simulink model "adc_to_10gbe"  (Simulink 7.4)
settings: Solver=ode45  StartTime=0.0  StopTime=200000  RelTol=1e-3
undefined symbols (not defined in the file): ROACH
libraries: xbsIndex_r4 x112, xps_library x77, casper_library_misc x6, xbsReplacements_r4 x3
(part 1 of 2)
settings Model: Creator=jkocz  LastModifiedBy=danny
settings OptimizationCC: InitFltsAndDblsToZero=on
settings DebuggingCC: SaveWithParameterizedLinksMsg=none  SignalResolutionControl=TryResolveAllWithWarning  MultiTaskDSMMsg=warning  MultiTaskCondExecSysMsg=none  StrictBusMsg=None
settings RTWCC: IncludeERTFirstTime=on
settings GRTTargetCC: TargetFcnLib=ansi_tfl_tmw.mat

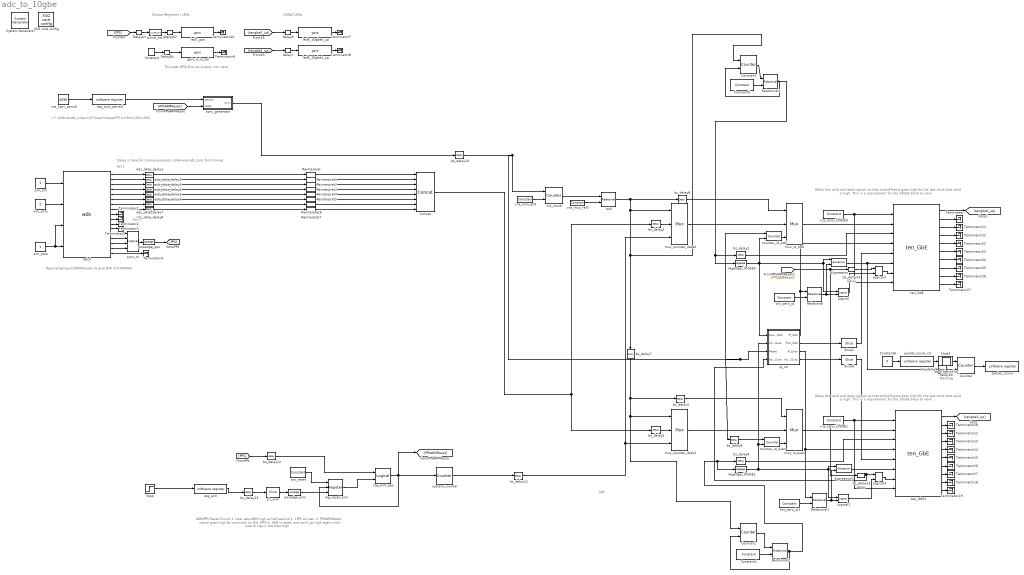
== system adc_to_10gbe ==
  note: left
  note: n * LCM(reoder_order=2)*(taps*clksperFFT=2*64=128)=256
  note: Pol 1
  note: Pol 2
  note: Real sampling at 800MSa/sec
      | to give B/W of 0-400MHz
  note: ARM/PPS Reset Circuit
      | 1. User sets ARM high at half-second
      | 2. 1PPS arrives.
      | 3. PPSARMReset signal goes high for one clock on the 1PPS
      | 4. ARM is reset, and won't go high again until user brings it low then high
  note: Delay is here for timing purposes:
      | otherwise adc_sync fails timing.
  note: Delay the valid and data signals so that
      | end-of-frame goes high for the last clock
      | that valid is high. This is a requirement for
      | the 10GbE block to work.
  note: Delay the valid and data signals so that
      | end-of-frame goes high for the last clock
      | that valid is high. This is a requirement for
      | the 10GbE block to work.
  note: This sets GPIO B as an output, not input
  note: Output Registers / LEDs
  note: 10GbE LEDa
  " System Generator" : xbsIndex_r4/ System Generator  Tag=genX  SystemSampleTime=-1  xilinxfamily=virtex2p  part=xc2vp50  speed=-7  package=ff1152  synthesis_tool=XST  clock_wrapper=Clock Enables  directory=./adc_to_10gbe_mod/sysgen  testbench=off  simulink_period=1  sysclk_period=5  dcm_input_clock_period=100  incr_netlist=off  trim_vbits=Everywhere in SubSystem  dbl_ovrd=According to Block Masks  core_generation=According to Block Masks  run_coregen=off  deprecated_control=off  eval_field=0  block_type=sysgen
      settings: block_version=10.1
  Concat : xbsIndex_r4/Concat  num_inputs=8  dbl_ovrd=off  block_type=concat
  Constant : xbsIndex_r4/Constant  arith_type=Boolean  const=0  n_bits=16  bin_pt=14  explicit_period=on  period=1  equ=P=C  opselect=C  inp2=PCIN>>17  opr=+  inp1=P  carry=CIN  dbl_ovrd=off  block_type=constant
      settings: block_version=11.4
  Constant1 : xbsIndex_r4/Constant  arith_type=Unsigned  const=1026  n_bits=11  bin_pt=0  explicit_period=off  period=1  equ=P=C  opselect=C  inp2=PCIN>>17  opr=+  inp1=P  carry=CIN  dbl_ovrd=off  block_type=constant
      settings: block_version=9.1.01
  Constant5 : xbsIndex_r4/Constant  arith_type=Unsigned  const=1026  n_bits=11  bin_pt=0  explicit_period=off  period=1  equ=P=C  opselect=C  inp2=PCIN>>17  opr=+  inp1=P  carry=CIN  dbl_ovrd=off  block_type=constant
      settings: block_version=9.1.01
  Constant6 : Constant  Value=0  OutDataType=sfix(16)  OutScaling=2^0
  Counter : xbsIndex_r4/Counter  cnt_type=Free Running  cnt_to=Inf  operation=Up  start_count=0  cnt_by_val=1  arith_type=Unsigned  n_bits=32  bin_pt=0  load_pin=off  rst=on  en=on  explicit_period=off  period=1  dbl_ovrd=off  use_behavioral_HDL=off  implementation=Fabric  use_rpm=on  block_type=counter
      settings: xl_area=[0, 0, 0, 0, 0, 0, 0]  block_version=10.1
  Counter1 : xbsIndex_r4/Counter  cnt_type=Free Running  cnt_to=1023  operation=Up  start_count=0  cnt_by_val=1  arith_type=Unsigned  n_bits=12  bin_pt=0  load_pin=off  rst=on  en=on  explicit_period=on  period=1  dbl_ovrd=off  use_behavioral_HDL=off  implementation=Fabric  use_rpm=on  block_type=counter
      settings: xl_area=[0, 0, 0, 0, 0, 0, 0]  block_version=9.1.01
  Counter3 : xbsIndex_r4/Counter  cnt_type=Free Running  cnt_to=1023  operation=Up  start_count=0  cnt_by_val=1  arith_type=Unsigned  n_bits=12  bin_pt=0  load_pin=off  rst=on  en=on  explicit_period=on  period=1  dbl_ovrd=off  use_behavioral_HDL=off  implementation=Fabric  use_rpm=on  block_type=counter
      settings: xl_area=[0, 0, 0, 0, 0, 0, 0]  block_version=9.1.01
  Delay{6..7,62..64} (5 alike) : xbsIndex_r4/Delay  en=off  latency=2  dbl_ovrd=off  reg_retiming=on  block_type=delay
  Expression : xbsIndex_r4/Expression  expression=a & ~b  align_bp=on  en=off  latency=0  precision=Full  arith_type=Unsigned  n_bits=8  bin_pt=2  dbl_ovrd=off  block_type=expr
      settings: xl_area=[0, 0, 0, 0, 0, 0, 0]  block_version=10.1
  Expression1 : xbsIndex_r4/Expression  expression=a & ~b  align_bp=on  en=off  latency=0  precision=Full  arith_type=Unsigned  n_bits=8  bin_pt=2  dbl_ovrd=off  block_type=expr
      settings: xl_area=[0, 0, 0, 0, 0, 0, 0]  block_version=10.1
  Logical : xbsIndex_r4/Logical  logical_function=AND  inputs=2  en=off  latency=0  precision=Full  arith_type=Unsigned  n_bits=8  bin_pt=2  align_bp=on  dbl_ovrd=off  block_type=logical
      settings: xl_area=[0, 0, 0, 0, 0, 0, 0]  block_version=10.1
  Logical1 : xbsIndex_r4/Logical  logical_function=AND  inputs=2  en=off  latency=0  precision=Full  arith_type=Unsigned  n_bits=8  bin_pt=2  align_bp=on  dbl_ovrd=off  block_type=logical
      settings: xl_area=[0, 0, 0, 0, 0, 0, 0]  block_version=10.1
  Logical3 : xbsIndex_r4/Logical  logical_function=OR  inputs=2  en=off  latency=0  precision=Full  arith_type=Unsigned  n_bits=8  bin_pt=2  align_bp=on  dbl_ovrd=off  block_type=logical
      settings: xl_area=[0, 0, 0, 0, 0, 0, 0]  block_version=10.1
  Logical4 : xbsIndex_r4/Logical  logical_function=OR  inputs=2  en=off  latency=0  precision=Full  arith_type=Unsigned  n_bits=8  bin_pt=2  align_bp=on  dbl_ovrd=off  block_type=logical
      settings: xl_area=[0, 0, 0, 0, 0, 0, 0]  block_version=10.1
  Reinterpret{,1..7} (8 alike) : xbsIndex_r4/Reinterpret  force_arith_type=on  arith_type=Unsigned  force_bin_pt=on  bin_pt=0  block_type=reinterpret
      Reinterpret settings: infoedit="Changes signal type without altering the binary representation.   You can changed the signal between signed and unsigned, and relocate the binary point.<br><br>Hardware notes: In hardware this block costs nothing.<br><br>Example:  Suppose the input is 6 bits wide, signed, with 2 fractional bits, and the output is forced to unsigned with 0 fractional bits.  Then an input of -2.0 (1110.00 in binary 2's complement) becomes an output of 56 (111000 in binary)."  block_version=10.1
      Reinterpret1 settings: infoedit="Changes signal type without altering the binary representation.   You can changed the signal between signed and unsigned, and relocate the binary point.<P><P>Hardware notes: In hardware this block costs nothing.<P><P>Example:  Suppose the input is 6 bits wide, signed, with 2 fractional bits, and the output is forced to unsigned with 0 fractional bits.  Then an input of -2.0 (1110.00 in binary 2's complement) becomes an output of 56 (111000 in binary)."  block_version=10.1
      Reinterpret2 settings: infoedit="Changes signal type without altering the binary representation.   You can changed the signal between signed and unsigned, and relocate the binary point.<P><P>Hardware notes: In hardware this block costs nothing.<P><P>Example:  Suppose the input is 6 bits wide, signed, with 2 fractional bits, and the output is forced to unsigned with 0 fractional bits.  Then an input of -2.0 (1110.00 in binary 2's complement) becomes an output of 56 (111000 in binary)."  block_version=10.1
      Reinterpret3 settings: infoedit="Changes signal type without altering the binary representation.   You can changed the signal between signed and unsigned, and relocate the binary point.<P><P>Hardware notes: In hardware this block costs nothing.<P><P>Example:  Suppose the input is 6 bits wide, signed, with 2 fractional bits, and the output is forced to unsigned with 0 fractional bits.  Then an input of -2.0 (1110.00 in binary 2's complement) becomes an output of 56 (111000 in binary)."  block_version=10.1
      Reinterpret4 settings: infoedit="Changes signal type without altering the binary representation.   You can changed the signal between signed and unsigned, and relocate the binary point.<P><P>Hardware notes: In hardware this block costs nothing.<P><P>Example:  Suppose the input is 6 bits wide, signed, with 2 fractional bits, and the output is forced to unsigned with 0 fractional bits.  Then an input of -2.0 (1110.00 in binary 2's complement) becomes an output of 56 (111000 in binary)."  block_version=10.1
      Reinterpret5 settings: infoedit="Changes signal type without altering the binary representation.   You can changed the signal between signed and unsigned, and relocate the binary point.<P><P>Hardware notes: In hardware this block costs nothing.<P><P>Example:  Suppose the input is 6 bits wide, signed, with 2 fractional bits, and the output is forced to unsigned with 0 fractional bits.  Then an input of -2.0 (1110.00 in binary 2's complement) becomes an output of 56 (111000 in binary)."  block_version=10.1
      Reinterpret6 settings: infoedit="Changes signal type without altering the binary representation.   You can changed the signal between signed and unsigned, and relocate the binary point.<P><P>Hardware notes: In hardware this block costs nothing.<P><P>Example:  Suppose the input is 6 bits wide, signed, with 2 fractional bits, and the output is forced to unsigned with 0 fractional bits.  Then an input of -2.0 (1110.00 in binary 2's complement) becomes an output of 56 (111000 in binary)."  block_version=10.1
      Reinterpret7 settings: infoedit="Changes signal type without altering the binary representation.   You can changed the signal between signed and unsigned, and relocate the binary point.<P><P>Hardware notes: In hardware this block costs nothing.<P><P>Example:  Suppose the input is 6 bits wide, signed, with 2 fractional bits, and the output is forced to unsigned with 0 fractional bits.  Then an input of -2.0 (1110.00 in binary 2's complement) becomes an output of 56 (111000 in binary)."  block_version=10.1
  Relational : xbsIndex_r4/Relational  mode=a=b  en=off  latency=1  dbl_ovrd=off  block_type=relational
      settings: xl_area=[0, 0, 0, 0, 0, 0, 0]  block_version=10.1
  Relational1 : xbsIndex_r4/Relational  mode=a=b  en=off  latency=1  dbl_ovrd=off  block_type=relational
      settings: xl_area=[0, 0, 0, 0, 0, 0, 0]  block_version=10.1
  Relational2 : xbsIndex_r4/Relational  mode=a!=b  en=off  latency=0  dbl_ovrd=off  block_type=relational
      settings: xl_area=[0, 0, 0, 0, 0, 0, 0]  block_version=9.1.01
  Relational5 : xbsIndex_r4/Relational  mode=a!=b  en=off  latency=0  dbl_ovrd=off  block_type=relational
      settings: xl_area=[0, 0, 0, 0, 0, 0, 0]  block_version=9.1.01
  Slice1 : xbsIndex_r4/Slice  nbits=16  boolean_output=off  mode=Lower Bit Location + Width  bit1=0  base1=MSB of Input  bit0=0  base0=LSB of Input  dbl_ovrd=off  block_type=slice
      settings: infoedit="Extracts a given range of bits from each input sample and presents it at the output.  The output type is ordinarily unsigned with binary point at zero, but can be Boolean when the slice is one bit wide.<P><P>Hardware notes: In hardware this block costs nothing."  block_version=10.1
  Slice3 : xbsIndex_r4/Slice  nbits=1  boolean_output=on  mode=Lower Bit Location + Width  bit1=0  base1=MSB of Input  bit0=0  base0=LSB of Input  dbl_ovrd=off  block_type=slice
      settings: infoedit="Extracts a given range of bits from each input sample and presents it at the output.  The output type is ordinarily unsigned with binary point at zero, but can be Boolean when the slice is one bit wide.<P><P>Hardware notes: In hardware this block costs nothing."  block_version=10.1
  Slice6 : xbsIndex_r4/Slice  nbits=16  boolean_output=off  mode=Lower Bit Location + Width  bit1=0  base1=MSB of Input  bit0=0  base0=LSB of Input  dbl_ovrd=off  block_type=slice
      settings: infoedit="Extracts a given range of bits from each input sample and presents it at the output.  The output type is ordinarily unsigned with binary point at zero, but can be Boolean when the slice is one bit wide.<P><P>Hardware notes: In hardware this block costs nothing."  block_version=10.1
  Step : Step  SampleTime=0
  Terminator{,1..5,7..9,11..28} (27 alike) : Terminator
  XSG core config : xps_library/XSG core config  Tag=xps:xsg  SystemSampleTime=-1  hw_sys=ROACH:sx95t  ibob_linux=off  clk_src=adc0_clk  iBOB_clk_src=adc0_clk  BEE2_ctrl_clk_src=sys_clk  BEE2_usr_clk_src=sys_clk  ROACH_clk_src=adc0_clk  CORR_clk_src=sys_clk  gpio_clk_io_group=iBOB:sma  gpio_clk_bit_index=0  clk_rate=100  sample_period=1  synthesis_tool=XST  mpc_type=powerpc440_ext
  adc0 : xps_library/adc  Tag=xps:adc  SystemSampleTime=-1  adc_brd=adc0  adc_clk_rate=800  adc_interleave=off  sample_period=1
  adc_data_delay{1..8} (8 alike) : xbsIndex_r4/Delay  en=off  latency=1  dbl_ovrd=off  reg_retiming=on  block_type=delay
      settings: xl_area=[0, 0, 0, 0, 0, 0, 0]  block_version=10.1
  bs_delay{1..2,4..5} (4 alike) : xbsIndex_r4/Delay  en=off  latency=1  dbl_ovrd=off  reg_retiming=off  block_type=delay
      settings: xl_area=[0, 0, 0, 0, 0, 0, 0]  block_version=10.1
  bs_delay{10..13} (4 alike) : xbsIndex_r4/Delay  en=off  latency=0  dbl_ovrd=off  reg_retiming=off  block_type=delay
      settings: xl_area=[0, 0, 0, 0, 0, 0, 0]  block_version=10.1
  bs_delay14 : xbsIndex_r4/Delay  en=off  latency=3  dbl_ovrd=off  reg_retiming=off  block_type=delay
      settings: xl_area=[0, 0, 0, 0, 0, 0, 0]  block_version=10.1
  bs_delay15 : xbsIndex_r4/Delay  en=off  latency=1027  dbl_ovrd=off  reg_retiming=off  block_type=delay
      settings: xl_area=[0, 0, 0, 0, 0, 0, 0]  block_version=10.1
  bs_delay3 : xbsIndex_r4/Delay  en=off  latency=2  dbl_ovrd=off  reg_retiming=off  block_type=delay
      settings: xl_area=[0, 0, 0, 0, 0, 0, 0]  block_version=10.1
  bs_delay6 : xbsIndex_r4/Delay  en=off  latency=4  dbl_ovrd=off  reg_retiming=off  block_type=delay
      settings: xl_area=[0, 0, 0, 0, 0, 0, 0]  block_version=10.1
  bs_delay7 : xbsIndex_r4/Delay  en=off  latency=1024  dbl_ovrd=off  reg_retiming=off  block_type=delay
      settings: xl_area=[0, 0, 0, 0, 0, 0, 0]  block_version=10.1
  bs_delay8 : xbsIndex_r4/Delay  en=off  latency=2  dbl_ovrd=off  reg_retiming=off  block_type=delay
      settings: xl_area=[0, 0, 0, 0, 0, 0, 0]  block_version=10.1
  bs_delay9 : xbsIndex_r4/Delay  en=off  latency=5  dbl_ovrd=off  reg_retiming=on  block_type=delay
      settings: xl_area=[0, 0, 0, 0, 0, 0, 0]  block_version=10.1
  cns_mux_en0 : xbsIndex_r4/Constant  arith_type=Boolean  const=1  n_bits=1  bin_pt=0  explicit_period=on  period=1  equ=P=C  opselect=C  inp2=PCIN>>17  opr=+  inp1=P  carry=CIN  dbl_ovrd=off  block_type=constant
      settings: block_version=10.1
  cns_mux_rel0 : xbsIndex_r4/Constant  arith_type=Unsigned  const=0  n_bits=11  bin_pt=0  explicit_period=on  period=1  equ=P=C  opselect=C  inp2=PCIN>>17  opr=+  inp1=P  carry=CIN  dbl_ovrd=off  block_type=constant
      settings: block_version=10.1
  cns_reset : xbsIndex_r4/Constant  arith_type=Boolean  const=1  n_bits=1  bin_pt=0  explicit_period=on  period=1  equ=P=C  opselect=C  inp2=PCIN>>17  opr=+  inp1=P  carry=CIN  dbl_ovrd=off  block_type=constant
      settings: block_version=10.1
  cns_sync_period : Constant  Value=4096  OutDataType=sfix(16)  OutScaling=2^0
  cns_zero_10GbE0 : xbsIndex_r4/Constant  arith_type=Boolean  const=0  n_bits=32  bin_pt=0  explicit_period=on  period=1  equ=P=C  opselect=C  inp2=PCIN>>17  opr=+  inp1=P  carry=CIN  dbl_ovrd=off  block_type=constant
      settings: block_version=10.1
  cns_zero_10GbE1 : xbsIndex_r4/Constant  arith_type=Boolean  const=0  n_bits=32  bin_pt=0  explicit_period=on  period=1  equ=P=C  opselect=C  inp2=PCIN>>17  opr=+  inp1=P  carry=CIN  dbl_ovrd=off  block_type=constant
      settings: block_version=10.1
  cns_zero_ip : xbsIndex_r4/Constant  arith_type=Unsigned  const=0  n_bits=32  bin_pt=0  explicit_period=on  period=1  equ=P=C  opselect=C  inp2=PCIN>>17  opr=+  inp1=P  carry=CIN  dbl_ovrd=off  block_type=constant
      settings: block_version=10.1
  cns_zero_ip1 : xbsIndex_r4/Constant  arith_type=Unsigned  const=0  n_bits=32  bin_pt=0  explicit_period=on  period=1  equ=P=C  opselect=C  inp2=PCIN>>17  opr=+  inp1=P  carry=CIN  dbl_ovrd=off  block_type=constant
      settings: block_version=10.1
  cnt_mux0 : xbsIndex_r4/Counter  cnt_type=Free Running  cnt_to=Inf  operation=Up  start_count=0  cnt_by_val=1  arith_type=Unsigned  n_bits=11  bin_pt=0  load_pin=off  rst=on  en=on  explicit_period=off  period=1  dbl_ovrd=off  use_behavioral_HDL=off  implementation=Fabric  use_rpm=on  block_type=counter
      settings: xl_area=[0, 0, 0, 0, 0, 0, 0]  block_version=10.1
  counter_id_even : xbsIndex_r4/Counter  cnt_type=Count Limited  cnt_to=16  operation=Up  start_count=2  cnt_by_val=2  arith_type=Unsigned  n_bits=64  bin_pt=0  load_pin=off  rst=on  en=on  explicit_period=off  period=1  dbl_ovrd=off  use_behavioral_HDL=off  implementation=Fabric  use_rpm=on  block_type=counter
      settings: xl_area=[0, 0, 0, 0, 0, 0, 0]  block_version=10.1
  counter_id_odd : xbsIndex_r4/Counter  cnt_type=Count Limited  cnt_to=15  operation=Up  start_count=1  cnt_by_val=2  arith_type=Unsigned  n_bits=64  bin_pt=0  load_pin=off  rst=on  en=on  explicit_period=off  period=1  dbl_ovrd=off  use_behavioral_HDL=off  implementation=Fabric  use_rpm=on  block_type=counter
      settings: xl_area=[0, 0, 0, 0, 0, 0, 0]  block_version=10.1
  gpio_b_io_sel : xps_library/gpio  Tag=xps:gpio  SystemSampleTime=-1  io_group=ROACH:gpiob_oe_n  io_dir=out  arith_type=Boolean  bitwidth=1  bin_pt=0  bit_index=0  sample_period=1  use_single_ended=off  use_ddr=off  reg_iob=on  reg_clk_phase=0  termination=None
      link override convert: arith_type=Boolean  n_bits=1  bin_pt=0
  ip_ctr : Subsystem  mask(ip_ctr){numcomputers=32}
      mask prompts: numcomputers "Num IPs (Must be power of 2)"
      mask init:
      | ip_ctr_init(gcb,...
      |     'numcomputers',numcomputers)
      settings: AttributesFormatString=IPs=32
  led5_10gbe0_up : xps_library/gpio  Tag=xps:gpio  SystemSampleTime=-1  io_group=ROACH:gpiob  io_dir=out  arith_type=Boolean  bitwidth=1  bin_pt=0  bit_index=5  sample_period=1  use_single_ended=off  use_ddr=off  reg_iob=on  reg_clk_phase=0  termination=None
      link override convert: arith_type=Boolean  n_bits=1  bin_pt=0
  led6_10gbe1_up : xps_library/gpio  Tag=xps:gpio  SystemSampleTime=-1  io_group=ROACH:gpiob  io_dir=out  arith_type=Boolean  bitwidth=1  bin_pt=0  bit_index=6  sample_period=1  use_single_ended=off  use_ddr=off  reg_iob=on  reg_clk_phase=0  termination=None
      link override convert: arith_type=Boolean  n_bits=1  bin_pt=0
  led7_pps : xps_library/gpio  Tag=xps:gpio  SystemSampleTime=-1  io_group=ROACH:gpiob  io_dir=out  arith_type=Boolean  bitwidth=1  bin_pt=0  bit_index=7  sample_period=1  use_single_ended=off  use_ddr=off  reg_iob=on  reg_clk_phase=0  termination=None
      link override convert: arith_type=Boolean  n_bits=1  bin_pt=0
  log_arm_pps : xbsIndex_r4/Logical  logical_function=AND  inputs=2  en=off  latency=0  precision=Full  arith_type=Unsigned  n_bits=8  bin_pt=2  align_bp=on  dbl_ovrd=off  block_type=logical
      settings: xl_area=[0, 0, 0, 0, 0, 0, 0]  block_version=10.1
  mux_counter_data0 : xbsIndex_r4/Mux  inputs=2  en=off  latency=1  precision=Full  arith_type="Signed  (2's comp)"  n_bits=8  bin_pt=2  quantization=Truncate  overflow=Wrap  dbl_ovrd=off  block_type=mux
      settings: xl_area=[0, 0, 0, 0, 0, 0, 0]  block_version=10.1
  mux_counter_data1 : xbsIndex_r4/Mux  inputs=2  en=off  latency=1  precision=Full  arith_type="Signed  (2's comp)"  n_bits=8  bin_pt=2  quantization=Truncate  overflow=Wrap  dbl_ovrd=off  block_type=mux
      settings: xl_area=[0, 0, 0, 0, 0, 0, 0]  block_version=10.1
  mux_id_even : xbsIndex_r4/Mux  inputs=2  en=off  latency=1  precision=Full  arith_type="Signed  (2's comp)"  n_bits=8  bin_pt=2  quantization=Truncate  overflow=Wrap  dbl_ovrd=off  block_type=mux
      settings: xl_area=[0, 0, 0, 0, 0, 0, 0]  block_version=10.1
  mux_id_odd : xbsIndex_r4/Mux  inputs=2  en=off  latency=1  precision=Full  arith_type="Signed  (2's comp)"  n_bits=8  bin_pt=2  quantization=Truncate  overflow=Wrap  dbl_ovrd=off  block_type=mux
      settings: xl_area=[0, 0, 0, 0, 0, 0, 0]  block_version=10.1
  negedge_10GbE0 : casper_library_misc/negedge  Tag=Rising Edge Detector  SystemSampleTime=-1
  negedge_10GbE1 : casper_library_misc/negedge  Tag=Rising Edge Detector  SystemSampleTime=-1
  packet_count : xps_library/software register  Tag=xps:sw_reg  SystemSampleTime=-1  io_dir=To Processor  arith_type=Unsigned  bitwidth=32  bin_pt=0  sample_period=1  gw_name=adc_to_10gbe_packet_count_user_data_in
      link override convert: arith_type=Unsigned  n_bits=32  bin_pt=0
  packet_count_rst : xps_library/software register  Tag=xps:sw_reg  SystemSampleTime=-1  io_dir=From Processor  arith_type=Unsigned  bitwidth=32  bin_pt=0  sample_period=1  gw_name=adc_to_10gbe_packet_count_rst_user_data_out
      link override adc_to_10gbe_mod_packet_count_rst_user_data_out: arith_type=Unsigned  n_bits=32  bin_pt=0  period=1
      link override adc_to_10gbe_packet_count_rst_user_data_out: arith_type=Unsigned  n_bits=32  bin_pt=0  period=1
  posedge_arm : casper_library_misc/posedge  Tag=Rising Edge Detector  SystemSampleTime=-1
  posedge_pps : casper_library_misc/posedge  Tag=Rising Edge Detector  SystemSampleTime=-1
  pulse_ext1 : casper_library_misc/pulse_ext  SystemSampleTime=-1  pulse_len=10000000
  reg_arm : xps_library/software register  Tag=xps:sw_reg  SystemSampleTime=-1  io_dir=From Processor  arith_type=Unsigned  bitwidth=32  bin_pt=0  sample_period=1  gw_name=adc_to_10gbe_reg_arm_user_data_out
      link override adc_to_10gbe_mod_reg_arm_user_data_out: arith_type=Unsigned  n_bits=32  bin_pt=0  period=1
      link override adc_to_10gbe_reg_arm_user_data_out: arith_type=Unsigned  n_bits=32  bin_pt=0  period=1
  reg_reset_arm : xbsIndex_r4/Register  init=0  rst=on  en=on  dbl_ovrd=off  block_type=register
      settings: xl_area=[0, 0, 0, 0, 0, 0, 0]  block_version=10.1
  reg_sync_period : xps_library/software register  Tag=xps:sw_reg  SystemSampleTime=-1  io_dir=From Processor  arith_type=Unsigned  bitwidth=32  bin_pt=0  sample_period=1  gw_name=adc_to_10gbe_reg_sync_period_user_data_out
      link override adc_to_10gbe_mod_reg_sync_period_user_data_out: arith_type=Unsigned  n_bits=32  bin_pt=0  period=1
      link override adc_to_10gbe_reg_sync_period_user_data_out: arith_type=Unsigned  n_bits=32  bin_pt=0  period=1
  rel0 : xbsIndex_r4/Relational  mode=a=b  en=off  latency=1  dbl_ovrd=off  block_type=relational
      settings: xl_area=[0, 0, 0, 0, 0, 0, 0]  block_version=10.1
  sim_cns : Constant  OutDataType=sfix(16)  OutScaling=2^0
  sim_cns1 : Constant  Value=2  OutDataType=sfix(16)  OutScaling=2^0
  sim_zero : Constant  OutDataType=sfix(16)  OutScaling=2^0
  slc_arm : xbsIndex_r4/Slice  nbits=1  boolean_output=on  mode=Lower Bit Location + Width  bit1=0  base1=MSB of Input  bit0=0  base0=LSB of Input  dbl_ovrd=off  block_type=slice
      settings: infoedit="Extracts a given range of bits from each input sample and presents it at the output.  The output type is ordinarily unsigned with binary point at zero, but can be Boolean when the slice is one bit wide.<P><P>Hardware notes: In hardware this block costs nothing."  block_version=10.1
  sync_generator : Subsystem
  sync_or : xbsIndex_r4/Logical  logical_function=OR  inputs=4  en=off  latency=1  precision=Full  arith_type=Unsigned  n_bits=8  bin_pt=2  align_bp=on  dbl_ovrd=off  block_type=logical
      settings: xl_area=[0, 0, 0, 0, 0, 0, 0]  block_version=10.1
  system_counter : xbsIndex_r4/Counter  cnt_type=Free Running  cnt_to=Inf  operation=Up  start_count=0  cnt_by_val=1  arith_type=Unsigned  n_bits=64  bin_pt=0  load_pin=off  rst=on  en=off  explicit_period=off  period=1  dbl_ovrd=off  use_behavioral_HDL=off  implementation=Fabric  use_rpm=on  block_type=counter
      settings: xl_area=[0, 0, 0, 0, 0, 0, 0]  block_version=10.1
  ten_GbE : xps_library/ten_GbE  Tag=xps:tengbe  SystemSampleTime=-1  port=ROACH:0  mac_lite=off  open_phy=off  show_param=on  pre_emph=2  swing=800  fab_en=off  fab_mac=0  fab_ip=0  fab_udp=0  fab_gate=0
  ten_GbE1 : xps_library/ten_GbE  Tag=xps:tengbe  SystemSampleTime=-1  port=ROACH:1  mac_lite=on  open_phy=off  show_param=on  pre_emph=2  swing=800  fab_en=off  fab_mac=0  fab_ip=0  fab_udp=0  fab_gate=0
  warn period bs_delay90 : xbsReplacements_r4/Warning  SystemSampleTime=-1  period=1
  wires:
  reg_sync_period/1 -> sync_generator/1(period)
  sim_zero/1 -> adc0/3, adc0/4
  adc0/1 -> adc_data_delay1/1
  sync_generator/1(sync) -> bs_delay10/1
  adc0/2 -> adc_data_delay2/1
  adc0/3 -> adc_data_delay3/1
  adc0/4 -> adc_data_delay4/1
  adc0/5 -> adc_data_delay5/1
  adc0/6 -> adc_data_delay6/1
  adc0/7 -> adc_data_delay7/1
  adc0/8 -> adc_data_delay8/1
  cns_sync_period/1 -> reg_sync_period/1
  adc0/13 -> sync_or/1
  adc0/14 -> sync_or/2
  adc0/15 -> sync_or/3
  adc0/16 -> sync_or/4
  sync_or/1 -> posedge_pps/1
  posedge_pps/1 -> [PPS]
  [PPSARMReset] -> sync_generator/2(reset)
  reg_arm/1 -> bs_delay13/1
  cns_reset/1 -> reg_reset_arm/1
  reg_reset_arm/1 -> log_arm_pps/2
  [PPS] -> bs_delay12/1
  log_arm_pps/1 -> reg_reset_arm/2, [PPSARMReset], system_counter/1
  slc_arm/1 -> posedge_arm/1
  posedge_arm/1 -> reg_reset_arm/3
  sim_cns/1 -> adc0/1
  sim_cns1/1 -> adc0/2
  adc_data_delay1/1 -> Reinterpret/1
  adc_data_delay2/1 -> Reinterpret1/1
  adc_data_delay3/1 -> Reinterpret2/1
  adc_data_delay4/1 -> Reinterpret3/1
  adc_data_delay5/1 -> Reinterpret4/1
  adc_data_delay6/1 -> Reinterpret5/1
  adc_data_delay7/1 -> Reinterpret6/1
  adc_data_delay8/1 -> Reinterpret7/1
  adc0/9 -> Terminator1/1
  adc0/10 -> Terminator2/1
  adc0/11 -> Terminator3/1
  adc0/12 -> Terminator5/1
  adc0/17 -> Terminator4/1
  Reinterpret/1 -> Concat/1
  Reinterpret1/1 -> Concat/2
  Reinterpret2/1 -> Concat/3
  Reinterpret3/1 -> Concat/4
  Reinterpret4/1 -> Concat/5
  Reinterpret5/1 -> Concat/6
  Reinterpret6/1 -> Concat/7
  Reinterpret7/1 -> Concat/8
  ten_GbE1/10 -> Terminator19/1
  ten_GbE1/9 -> Terminator18/1
  ten_GbE1/8 -> Terminator17/1
  ten_GbE1/7 -> Terminator16/1
  ten_GbE1/6 -> Terminator15/1
  ten_GbE1/5 -> Terminator14/1
  ten_GbE1/4 -> Terminator13/1
  ten_GbE1/3 -> Terminator12/1
  ten_GbE1/2 -> Terminator28/1
  ten_GbE/10 -> Terminator27/1
  ten_GbE/9 -> Terminator26/1
  ten_GbE/8 -> Terminator25/1
  ten_GbE/7 -> Terminator24/1
  ten_GbE/6 -> Terminator23/1
  ten_GbE/5 -> Terminator22/1
  ten_GbE/4 -> Terminator21/1
  ten_GbE/3 -> Terminator11/1
  ten_GbE/2 -> Terminator/1
  ten_GbE/1 -> [tengbe0_up]
  cns_zero_10GbE0/1 -> ten_GbE/8, ten_GbE/1
  mux_counter_data0/1 -> mux_id_odd/2
  cnt_mux0/1 -> rel0/1
  cns_mux_en0/1 -> cnt_mux0/2
  negedge_10GbE0/1 -> Logical/1, Expression/1, counter_id_odd/2, ip_ctr/1(Count_Odd)
  cns_mux_rel0/1 -> rel0/2
  rel0/1 -> mux_counter_data0/1, bs_delay7/1, Counter3/1, bs_delay8/1
  bs_delay1/1 -> ten_GbE/3
  mux_id_odd/1 -> ten_GbE/2
  bs_delay2/1 -> mux_counter_data0/2
  ten_GbE1/1 -> [tengbe1_up]
  cns_zero_10GbE1/1 -> ten_GbE1/8, ten_GbE1/1
  mux_counter_data1/1 -> mux_id_even/2
  negedge_10GbE1/1 -> Logical1/1, Expression1/1, counter_id_even/2, ip_ctr/2(Count_Even)
  bs_delay4/1 -> ten_GbE1/3
  mux_id_even/1 -> ten_GbE1/2
  bs_delay5/1 -> mux_counter_data1/2
  bs_delay7/1 -> mux_counter_data1/1, Counter1/1, bs_delay3/1
  cns_zero_ip/1 -> Relational/2
  Logical/1 -> Logical3/2
  Relational/1 -> Logical/2, Expression/2
  Expression/1 -> bs_delay9/1, ten_GbE/6
  Relational1/1 -> Logical1/2, Expression1/2
  Expression1/1 -> ten_GbE1/6
  cns_zero_ip1/1 -> Relational1/2
  ip_ctr/2(Port_Odd) -> Slice1/1
  Slice1/1 -> ten_GbE/5
  Slice6/1 -> ten_GbE1/5
  ip_ctr/4(Port_Even) -> Slice6/1
  ip_ctr/1(IP_Odd) -> Relational/1, ten_GbE/4
  bs_delay8/1 -> mux_id_odd/1
  counter_id_odd/1 -> mux_id_odd/3
  bs_delay3/1 -> mux_id_even/1
  counter_id_even/1 -> mux_id_even/3
  ip_ctr/3(IP_Even) -> Relational1/1, ten_GbE1/4
  bs_delay6/1 -> counter_id_even/1
  Counter/1 -> packet_count/1
  Constant6/1 -> packet_count_rst/1
  packet_count_rst/1 -> Slice3/1
  Slice3/1 -> Counter/1
  bs_delay9/1 -> Counter/2
  system_counter/1 -> bs_delay11/1
  bs_delay10/1 -> counter_id_odd/1, bs_delay6/1, ip_ctr/3(Reset), cnt_mux0/1
  bs_delay11/1 -> mux_counter_data1/3, mux_counter_data0/3
  Relational5/1 -> Counter3/2, bs_delay1/1, negedge_10GbE0/1
  Constant5/1 -> Relational5/2
  Counter3/1 -> Relational5/1
  Step/1 -> reg_arm/1
  Concat/1 -> bs_delay2/1, bs_delay5/1
  [PPSARMReset] -> bs_delay14/1, bs_delay15/1
  Logical3/1 -> ten_GbE/7
  bs_delay14/1 -> Logical3/1
  bs_delay15/1 -> Logical4/1, ip_ctr/4(Reset_Even)
  Logical1/1 -> Logical4/2
  Logical4/1 -> ten_GbE1/7
  Relational2/1 -> Counter1/2, negedge_10GbE1/1, bs_delay4/1
  Constant1/1 -> Relational2/2
  Counter1/1 -> Relational2/1
  bs_delay12/1 -> log_arm_pps/1
  bs_delay13/1 -> slc_arm/1
  gpio_b_io_sel/1 -> Terminator9/1
  Constant/1 -> Delay64/1
  Delay64/1 -> gpio_b_io_sel/1
  led7_pps/1 -> Terminator20/1
  pulse_ext1/1 -> Delay62/1
  [PPS] -> Delay63/1
  Delay62/1 -> led7_pps/1
  Delay63/1 -> pulse_ext1/1
  led5_10gbe0_up/1 -> Terminator7/1
  [tengbe0_up] -> Delay6/1
  Delay6/1 -> led5_10gbe0_up/1
  led6_10gbe1_up/1 -> Terminator8/1
  [tengbe1_up] -> Delay7/1
  Delay7/1 -> led6_10gbe1_up/1
